simulink model "test_pi_flocking_gazebo"  (R2023b)
settings: Solver=FixedStepAuto  StartTime=0.0  StopTime=inf  RelTol=1e-3
values from neighbouring files (symbols this model uses):
  d_prime = 1    [main_flock3.m]    (also in main_flock4.m; params_flocking_ros.m)
  epsilon = 0.1    [main_flock3.m]    (also in main_flock4.m; params_flocking_ros.m)
  h = 0.2    [main_flock3.m]    (also in main_flock4.m; params_flocking_ros.m)
  R = 0.15    [main_flock3.m]    (also in main_flock4.m; params_flocking_ros.m)
  vxobs = 0    [main_flock3.m]    (also in main_flock4.m)
  vyobs = 0    [main_flock3.m]    (also in main_flock4.m)
  vzobs = 0    [main_flock3.m]    (also in main_flock4.m)
  xobs = 0.75    [main_flock3.m]    (also in main_flock4.m)
  yobs = -0.25    [main_flock3.m]    (also in main_flock4.m)
  zobs = 1.7    [main_flock3.m]    (also in main_flock4.m)
undefined symbols (not defined in the file or in its folder): angular, DiscIntNeverNeededParam, linear
libraries: ros2lib x14, simulink x4, robotcorelib x4
(part 1 of 2)
settings Model: Creator=johvany  LastModifiedBy=jonatan_alvarez
settings OptimizationCC: EnhancedBackFolding=on  PassReuseOutputArgsThreshold=0  ZeroExternalMemoryAtStartup=off  ZeroInternalMemoryAtStartup=off  MaxStackSize=64  OptimizeBlockOrder=speed  DifferentSizesBufferReuse=on  OptimizationCustomize=off
settings DebuggingCC: ParameterTunabilityLossMsg=error
settings HardwareCC: ProdBitPerLong=64  ProdHWDeviceType=Intel->x86-64 (Linux 64)  UseEmbeddedCoderFeatures=off
settings SFSimCC: MATLABDynamicMemAlloc=off
settings RTWCC: Description=Embedded Coder  SystemTargetFile=ert.tlc  HardwareBoard=Robot Operating System 2 (ROS 2)  TLCOptions="-aInlineSetEventsForThisBaseRateFcn=TLC_FALSE -aSuppressMultiTaskScheduler=TLC_FALSE  -aRateBasedStepFcn=0"  TemplateMakefile=ert_default_tmf  Toolchain=Colcon Tools  TargetLang=C++
settings CodeAppCC: ForceParamTrailComments=on  OperatorAnnotations=on
settings ERTTargetCC: ERTCustomFileBanners=off  CodeInterfacePackaging=C++ class  SupportContinuousTime=on  SupportNonInlinedSFcns=on  RemoveResetFunc=off  ModelStepFunctionPrototypeControlCompliant=off  RootIOFormat=Structure reference

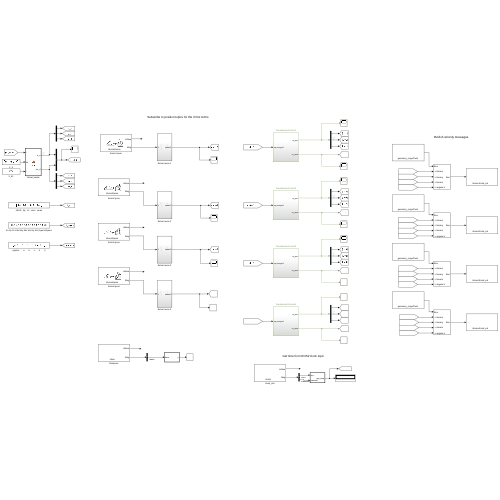
[thumbnail: Simulink's stored preview of the top-level diagram]
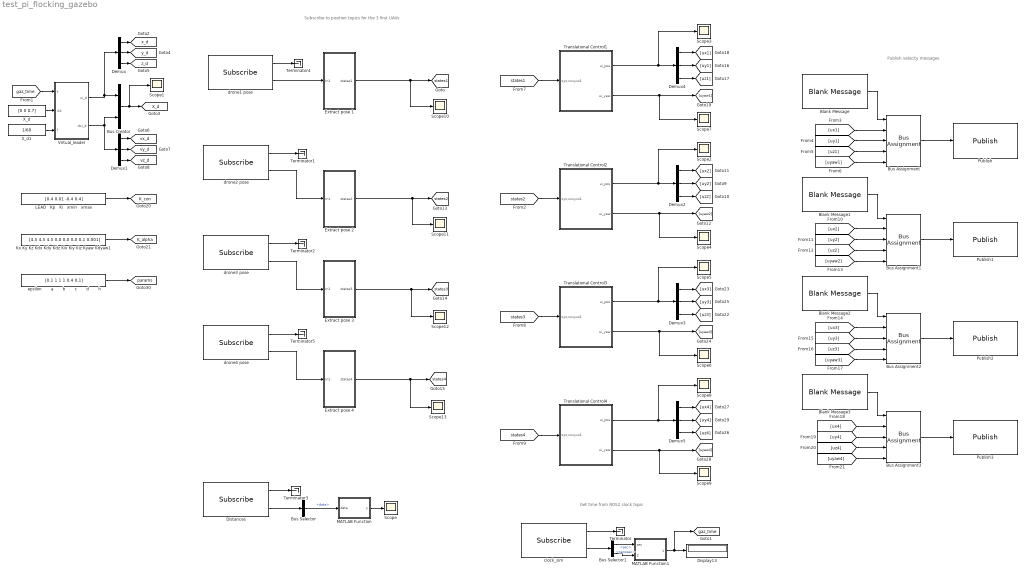
== system test_pi_flocking_gazebo ==
  note: Publish velocity messages
  note: Subscribe to position topics for the 3 first UAVs
  note: Get time from ROS2 clock topic
  Blank Message{,1..3} (4 alike) : ros2lib/Blank Message  messageClass=Message  entityType=geometry_msgs/Twist  messageType=geometry_msgs/Twist  SampleTime=inf
  Bus Assignment{,1..3} (4 alike) : BusAssignment  AssignedSignals=linear.x,linear.y,linear.z,angular.z
  Bus Creator : BusCreator  Inputs=2
  Bus Selector : BusSelector  OutputSignals=data
  Bus Selector1 : BusSelector  OutputSignals=clock.sec,clock.nanosec
  Demux{,1..5} (6 alike) : Demux  Outputs=3
  Display13 : Display
      settings: Decimation=4
  Distances : ros2lib/Subscribe  topicSource=Select from ROS network  topic=/dists  messageType=std_msgs/Float32MultiArray  sampleTime=-1  QOSHistory=Keep last  QOSDepth=1  QOSReliability=Reliable  QOSDurability=Volatile
  Extract pose 1 : Subsystem
  Extract pose 2 : Subsystem
  Extract pose 3 : Subsystem
  Extract pose 4 : Subsystem
  Kx Ky Kz Kdx Kdy Kdz Kix Kiy Kiz Kyaw Kdyaw1 : Constant  Value=[4.5 4.5 4.5 0.0 0.0 0.0 0.1 0.001]
  LEAD   Kp   Ki   xmin   xmax : Constant  Value=[0.4 0.01 -0.4 0.4]
  MATLAB Function : MATLAB Function  TreatAsAtomicUnit=on
  MATLAB Function1 : MATLAB Function  TreatAsAtomicUnit=on
  Publish : ros2lib/Publish  topicSource=Select from ROS network  topic=/drone1/cmd_vel  messageType=geometry_msgs/Twist  QOSHistory=Keep last  QOSDepth=1  QOSReliability=Reliable  QOSDurability=Volatile
  Publish1 : ros2lib/Publish  topicSource=Select from ROS network  topic=/drone2/cmd_vel  messageType=geometry_msgs/Twist  QOSHistory=Keep last  QOSDepth=1  QOSReliability=Reliable  QOSDurability=Volatile
  Publish2 : ros2lib/Publish  topicSource=Select from ROS network  topic=/drone3/cmd_vel  messageType=geometry_msgs/Twist  QOSHistory=Keep last  QOSDepth=1  QOSReliability=Reliable  QOSDurability=Volatile
  Publish3 : ros2lib/Publish  topicSource=Select from ROS network  topic=/drone4/cmd_vel  messageType=geometry_msgs/Twist  QOSHistory=Keep last  QOSDepth=1  QOSReliability=Reliable  QOSDurability=Volatile
  Scope{,1..13} (14 alike) : Scope
  Terminator{,1..5} (6 alike) : Terminator
  Translational Control1 : Subsystem
  Translational Control2 : Subsystem
  Translational Control3 : Subsystem
  Translational Control4 : Subsystem
  Virtual_leader : MATLAB Function  TreatAsAtomicUnit=on
  X_d : Constant  Value=[0 0 0.7]
  X_d1 : Constant  Value=1/60
  clock_sim : ros2lib/Subscribe  topicSource=Select from ROS network  topic=/clock  messageType=rosgraph_msgs/Clock  sampleTime=-1  QOSHistory=Keep last  QOSDepth=1  QOSReliability=Reliable  QOSDurability=Volatile
  drone1 pose : ros2lib/Subscribe  topicSource=Select from ROS network  topic=/drone1/pose  messageType=geometry_msgs/PoseStamped  sampleTime=-1  QOSHistory=Keep last  QOSDepth=1  QOSReliability=Reliable  QOSDurability=Volatile
  drone2 pose : ros2lib/Subscribe  topicSource=Select from ROS network  topic=/drone2/pose  messageType=geometry_msgs/PoseStamped  sampleTime=-1  QOSHistory=Keep last  QOSDepth=1  QOSReliability=Reliable  QOSDurability=Volatile
  drone3 pose : ros2lib/Subscribe  topicSource=Select from ROS network  topic=/drone3/pose  messageType=geometry_msgs/PoseStamped  sampleTime=-1  QOSHistory=Keep last  QOSDepth=1  QOSReliability=Reliable  QOSDurability=Volatile
  drone4 pose : ros2lib/Subscribe  topicSource=Select from ROS network  topic=/drone4/pose  messageType=geometry_msgs/PoseStamped  sampleTime=-1  QOSHistory=Keep last  QOSDepth=1  QOSReliability=Reliable  QOSDurability=Volatile
  epsilon       a       b       c       d       h : Constant  Value=[0.1 1 1 1 0.4 0.1]
  tag scope: K_alpha=global, K_con=global, X_d=global, gaz_time=global, params=global, states1=global, states2=global, states3=global, states4=global, vx_d=global, vy_d=global, vz_d=global, x_d=global, y_d=global, z_d=global
  wires:
  clock_sim/1 -> Terminator/1
  drone2 pose/2 -> Extract pose 2/1(In1)
  drone2 pose/1 -> Terminator1/1
  drone3 pose/2 -> Extract pose 3/1(In1)
  drone3 pose/1 -> Terminator2/1
  Blank Message/1 -> Bus Assignment/1
  Bus Assignment/1 -> Publish/1
  Blank Message1/1 -> Bus Assignment1/1
  Bus Assignment1/1 -> Publish1/1
  Blank Message2/1 -> Bus Assignment2/1
  Bus Assignment2/1 -> Publish2/1
  Blank Message3/1 -> Bus Assignment3/1
  Bus Assignment3/1 -> Publish3/1
  Distances/1 -> Terminator3/1
  Distances/2 -> Bus Selector/1
  Bus Selector/1 -> MATLAB Function/1(data)  "<data>"
  MATLAB Function/1(y) -> Scope/1
  clock_sim/2 -> Bus Selector1/1
  Bus Selector1/1 -> MATLAB Function1/1(sec)  "<sec>"
  Bus Selector1/2 -> MATLAB Function1/2(nanosec)  "<nanosec>"
  Demux1/1 -> [vx_d]
  Demux1/3 -> [vz_d]
  Demux/1 -> [x_d]
  Demux/2 -> [y_d]
  Virtual_leader/2(dxi_d) -> Bus Creator/2, Demux1/1
  Bus Creator/1 -> Scope1/1, [X_d]
  Demux1/2 -> [vy_d]
  [gaz_time] -> Virtual_leader/1(t)
  Demux/3 -> [z_d]
  Virtual_leader/1(xi_d) -> Bus Creator/1, Demux/1
  drone1 pose/1 -> Terminator4/1
  drone1 pose/2 -> Extract pose 1/1(In1)
  MATLAB Function1/1(gaz_time) -> [gaz_time], Display13/1
  Extract pose 1/1(states1) -> Scope10/1, [states1]
  [ux1] -> Bus Assignment/2
  [uy1] -> Bus Assignment/3
  [uz1] -> Bus Assignment/4
  [uyaw1] -> Bus Assignment/5
  X_d/1 -> Virtual_leader/2(Xd)
  Extract pose 2/1(states2) -> Scope11/1, [states2]
  Extract pose 3/1(states3) -> Scope12/1, [states3]
  drone4 pose/2 -> Extract pose 4/1(In1)
  drone4 pose/1 -> Terminator5/1
  Extract pose 4/1(states4) -> Scope13/1, [states4]
  [ux2] -> Bus Assignment1/2
  [uy2] -> Bus Assignment1/3
  [uz2] -> Bus Assignment1/4
  [uyaw2] -> Bus Assignment1/5
  [uy3] -> Bus Assignment2/3
  [uyaw3] -> Bus Assignment2/5
  [uz3] -> Bus Assignment2/4
  [ux3] -> Bus Assignment2/2
  [ux4] -> Bus Assignment3/2
  [uy4] -> Bus Assignment3/3
  [uz4] -> Bus Assignment3/4
  [uyaw4] -> Bus Assignment3/5
  Translational Control1/2(ui_yaw) -> [uyaw1], Scope7/1
  Demux4/2 -> [uy1]
  Demux4/3 -> [uz1]
  [states1] -> Translational Control1/1(xyz,vxvyvz1)
  Translational Control1/1(ui_pos) -> Scope3/1, Demux4/1
  Demux4/1 -> [ux1]
  LEAD   Kp   Ki   xmin   xmax/1 -> [K_con]
  Kx Ky Kz Kdx Kdy Kdz Kix Kiy Kiz Kyaw Kdyaw1/1 -> [K_alpha]
  Demux2/1 -> [ux2]
  Translational Control2/1(ui_pos) -> Demux2/1, Scope2/1
  [states2] -> Translational Control2/1(xyz,vxvyvz1)
  Demux2/3 -> [uz2]
  Demux2/2 -> [uy2]
  Translational Control2/2(ui_yaw) -> Scope4/1, [uyaw2]
  Translational Control3/2(ui_yaw) -> [uyaw3], Scope6/1
  Demux3/2 -> [uy3]
  Demux3/3 -> [uz3]
  [states3] -> Translational Control3/1(xyz,vxvyvz1)
  Translational Control3/1(ui_pos) -> Scope5/1, Demux3/1
  Demux3/1 -> [ux3]
  Demux5/1 -> [ux4]
  Translational Control4/1(ui_pos) -> Demux5/1, Scope8/1
  [states4] -> Translational Control4/1(xyz,vxvyvz1)
  Demux5/3 -> [uz4]
  Demux5/2 -> [uy4]
  Translational Control4/2(ui_yaw) -> Scope9/1, [uyaw4]
  epsilon       a       b       c       d       h/1 -> [params]
  X_d1/1 -> Virtual_leader/3(f)

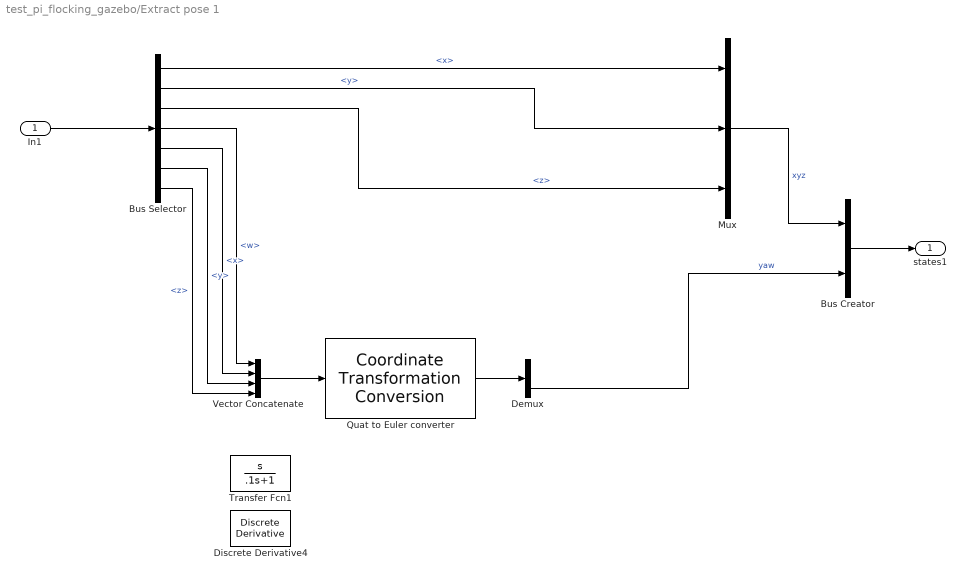
== system test_pi_flocking_gazebo/Extract pose 1 ==
  In1 : Inport
  Bus Creator : BusCreator  Inputs=2
  Bus Selector : BusSelector  OutputSignals=pose.position.x,pose.position.y,pose.position.z,pose.orientation.w,pose.orientation.x,pose.orientation.y,pose.orientation.z
  Demux : Demux  Outputs=3
  Discrete Derivative4 : simulink/Discrete/Discrete Derivative  gainval=1.0  ICPrevScaledInput=0.0  OutMin=[]  OutMax=[]  OutDataType=fixdt(1, 16)  OutScaling=2^-10  DoSatur=off
  Mux : Mux  Inputs=3
  Quat to Euler converter : robotcorelib/Coordinate Transformation Conversion  InputRepresentation=Quaternion  InputEulerSequence=ZYX  ShowTrVecInputPort=on  OutputRepresentation=Euler Angles  OutputEulerSequence=XYZ  ShowTrVecOutputPort=on  SimulateUsing=Interpreted execution
      settings: LibrarySourceBlock=roslib/Utilities/Coordinate Transformation Conversion
  Transfer Fcn1 : TransferFcn  Numerator=[1 0]  Denominator=[.1 1]
  Vector Concatenate : Concatenate  NumInputs=4
  states1 : Outport
  wires:
  Bus Selector/5 -> Vector Concatenate/2  "<x>"
  Quat to Euler converter/1 -> Demux/1
  Bus Selector/6 -> Vector Concatenate/3  "<y>"
  Bus Selector/1 -> Mux/1  "<x>"
  Bus Selector/7 -> Vector Concatenate/4  "<z>"
  Vector Concatenate/1 -> Quat to Euler converter/1
  In1/1 -> Bus Selector/1
  Bus Selector/4 -> Vector Concatenate/1  "<w>"
  Bus Selector/2 -> Mux/2  "<y>"
  Bus Selector/3 -> Mux/3  "<z>"
  Demux/3 -> Bus Creator/2  "yaw"
  Mux/1 -> Bus Creator/1  "xyz"
  Bus Creator/1 -> states1/1

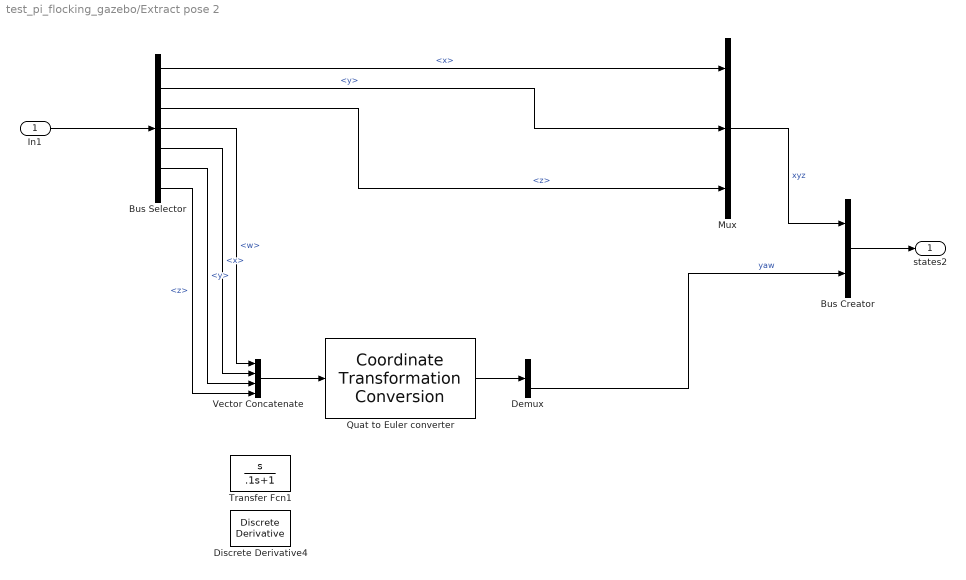
== system test_pi_flocking_gazebo/Extract pose 2 ==
  In1 : Inport
  Bus Creator : BusCreator  Inputs=2
  Bus Selector : BusSelector  OutputSignals=pose.position.x,pose.position.y,pose.position.z,pose.orientation.w,pose.orientation.x,pose.orientation.y,pose.orientation.z
  Demux : Demux  Outputs=3
  Discrete Derivative4 : simulink/Discrete/Discrete Derivative  gainval=1.0  ICPrevScaledInput=0.0  OutMin=[]  OutMax=[]  OutDataType=fixdt(1, 16)  OutScaling=2^-10  DoSatur=off
  Mux : Mux  Inputs=3
  Quat to Euler converter : robotcorelib/Coordinate Transformation Conversion  InputRepresentation=Quaternion  InputEulerSequence=ZYX  ShowTrVecInputPort=on  OutputRepresentation=Euler Angles  OutputEulerSequence=XYZ  ShowTrVecOutputPort=on  SimulateUsing=Interpreted execution
      settings: LibrarySourceBlock=roslib/Utilities/Coordinate Transformation Conversion
  Transfer Fcn1 : TransferFcn  Numerator=[1 0]  Denominator=[.1 1]
  Vector Concatenate : Concatenate  NumInputs=4
  states2 : Outport
  wires:
  Bus Creator/1 -> states2/1
  Mux/1 -> Bus Creator/1  "xyz"
  Demux/3 -> Bus Creator/2  "yaw"
  Bus Selector/3 -> Mux/3  "<z>"
  Bus Selector/2 -> Mux/2  "<y>"
  Bus Selector/4 -> Vector Concatenate/1  "<w>"
  In1/1 -> Bus Selector/1
  Vector Concatenate/1 -> Quat to Euler converter/1
  Bus Selector/7 -> Vector Concatenate/4  "<z>"
  Bus Selector/1 -> Mux/1  "<x>"
  Bus Selector/6 -> Vector Concatenate/3  "<y>"
  Quat to Euler converter/1 -> Demux/1
  Bus Selector/5 -> Vector Concatenate/2  "<x>"

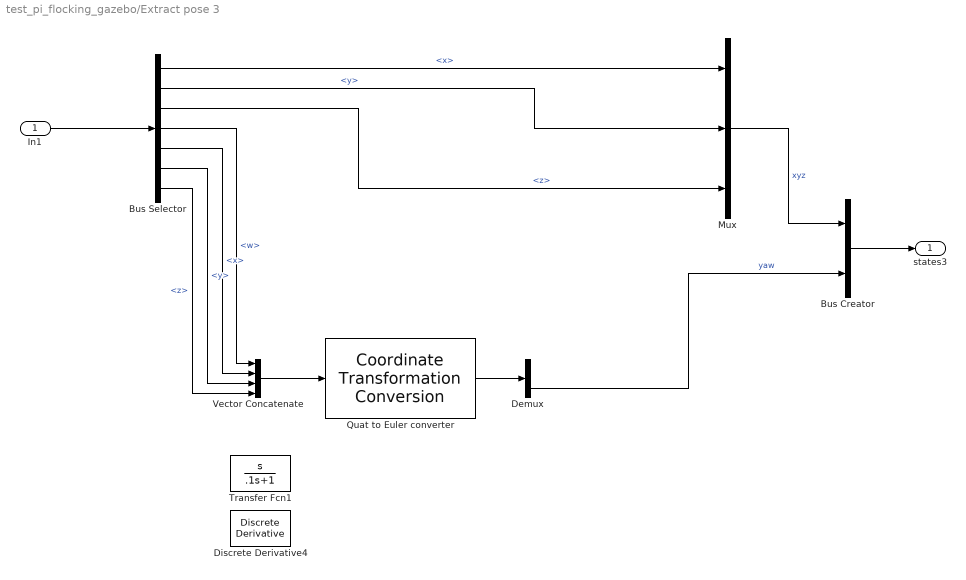
== system test_pi_flocking_gazebo/Extract pose 3 ==
  In1 : Inport
  Bus Creator : BusCreator  Inputs=2
  Bus Selector : BusSelector  OutputSignals=pose.position.x,pose.position.y,pose.position.z,pose.orientation.w,pose.orientation.x,pose.orientation.y,pose.orientation.z
  Demux : Demux  Outputs=3
  Discrete Derivative4 : simulink/Discrete/Discrete Derivative  gainval=1.0  ICPrevScaledInput=0.0  OutMin=[]  OutMax=[]  OutDataType=fixdt(1, 16)  OutScaling=2^-10  DoSatur=off
  Mux : Mux  Inputs=3
  Quat to Euler converter : robotcorelib/Coordinate Transformation Conversion  InputRepresentation=Quaternion  InputEulerSequence=ZYX  ShowTrVecInputPort=on  OutputRepresentation=Euler Angles  OutputEulerSequence=XYZ  ShowTrVecOutputPort=on  SimulateUsing=Interpreted execution
      settings: LibrarySourceBlock=roslib/Utilities/Coordinate Transformation Conversion
  Transfer Fcn1 : TransferFcn  Numerator=[1 0]  Denominator=[.1 1]
  Vector Concatenate : Concatenate  NumInputs=4
  states3 : Outport
  wires:
  Bus Selector/5 -> Vector Concatenate/2  "<x>"
  Quat to Euler converter/1 -> Demux/1
  Bus Selector/6 -> Vector Concatenate/3  "<y>"
  Bus Selector/1 -> Mux/1  "<x>"
  Bus Selector/7 -> Vector Concatenate/4  "<z>"
  Vector Concatenate/1 -> Quat to Euler converter/1
  In1/1 -> Bus Selector/1
  Bus Selector/4 -> Vector Concatenate/1  "<w>"
  Bus Selector/2 -> Mux/2  "<y>"
  Bus Selector/3 -> Mux/3  "<z>"
  Demux/3 -> Bus Creator/2  "yaw"
  Mux/1 -> Bus Creator/1  "xyz"
  Bus Creator/1 -> states3/1

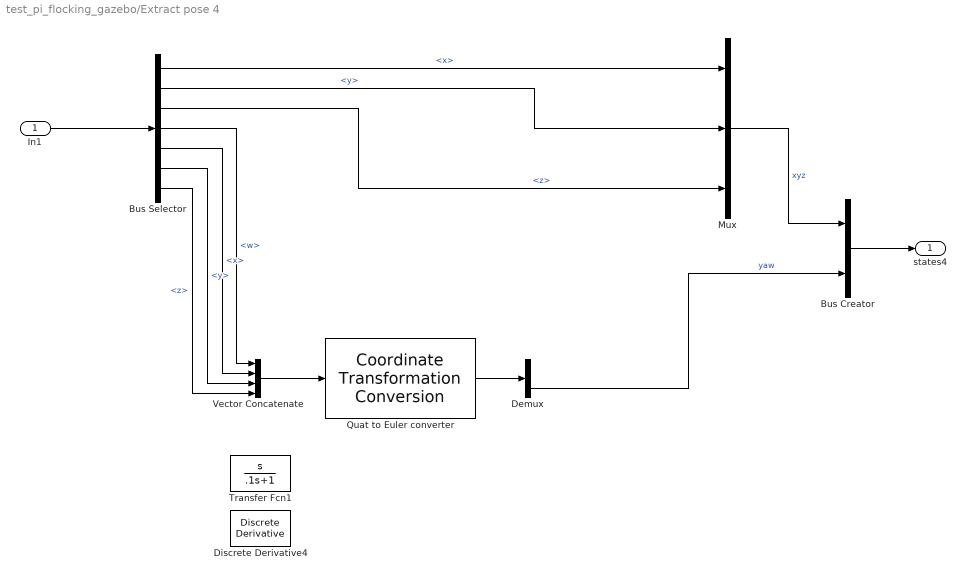
== system test_pi_flocking_gazebo/Extract pose 4 ==
  In1 : Inport
  Bus Creator : BusCreator  Inputs=2
  Bus Selector : BusSelector  OutputSignals=pose.position.x,pose.position.y,pose.position.z,pose.orientation.w,pose.orientation.x,pose.orientation.y,pose.orientation.z
  Demux : Demux  Outputs=3
  Discrete Derivative4 : simulink/Discrete/Discrete Derivative  gainval=1.0  ICPrevScaledInput=0.0  OutMin=[]  OutMax=[]  OutDataType=fixdt(1, 16)  OutScaling=2^-10  DoSatur=off
  Mux : Mux  Inputs=3
  Quat to Euler converter : robotcorelib/Coordinate Transformation Conversion  InputRepresentation=Quaternion  InputEulerSequence=ZYX  ShowTrVecInputPort=on  OutputRepresentation=Euler Angles  OutputEulerSequence=XYZ  ShowTrVecOutputPort=on  SimulateUsing=Interpreted execution
      settings: LibrarySourceBlock=roslib/Utilities/Coordinate Transformation Conversion
  Transfer Fcn1 : TransferFcn  Numerator=[1 0]  Denominator=[.1 1]
  Vector Concatenate : Concatenate  NumInputs=4
  states4 : Outport
  wires:
  Bus Creator/1 -> states4/1
  Mux/1 -> Bus Creator/1  "xyz"
  Demux/3 -> Bus Creator/2  "yaw"
  Bus Selector/3 -> Mux/3  "<z>"
  Bus Selector/2 -> Mux/2  "<y>"
  Bus Selector/4 -> Vector Concatenate/1  "<w>"
  In1/1 -> Bus Selector/1
  Vector Concatenate/1 -> Quat to Euler converter/1
  Bus Selector/7 -> Vector Concatenate/4  "<z>"
  Bus Selector/1 -> Mux/1  "<x>"
  Bus Selector/6 -> Vector Concatenate/3  "<y>"
  Quat to Euler converter/1 -> Demux/1
  Bus Selector/5 -> Vector Concatenate/2  "<x>"

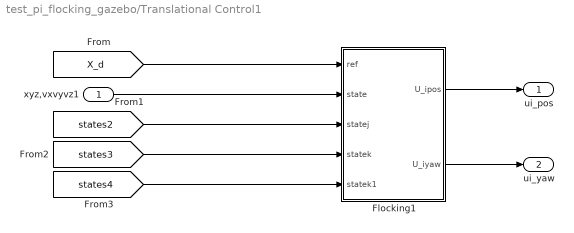
== system test_pi_flocking_gazebo/Translational Control1 ==
  xyz,vxvyvz1 : Inport
  Flocking1 : Subsystem
  ui_pos : Outport  VectorParamsAs1DForOutWhenUnconnected=off
  ui_yaw : Outport  Port=2  VectorParamsAs1DForOutWhenUnconnected=off
  wires:
  [X_d] -> Flocking1/1(ref)
  xyz,vxvyvz1/1 -> Flocking1/2(state)
  [states2] -> Flocking1/3(statej)
  [states3] -> Flocking1/4(statek)
  [states4] -> Flocking1/5(statek1)
  Flocking1/1(U_ipos) -> ui_pos/1
  Flocking1/2(U_iyaw) -> ui_yaw/1

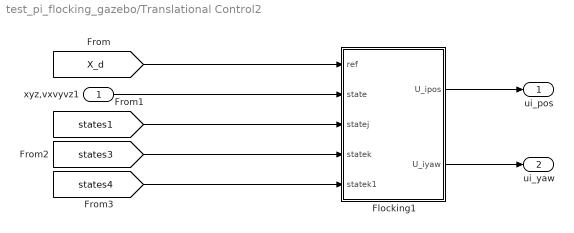
== system test_pi_flocking_gazebo/Translational Control2 ==
  xyz,vxvyvz1 : Inport
  Flocking1 : Subsystem
  ui_pos : Outport  VectorParamsAs1DForOutWhenUnconnected=off
  ui_yaw : Outport  Port=2  VectorParamsAs1DForOutWhenUnconnected=off
  wires:
  Flocking1/2(U_iyaw) -> ui_yaw/1
  Flocking1/1(U_ipos) -> ui_pos/1
  [states4] -> Flocking1/5(statek1)
  [states3] -> Flocking1/4(statek)
  [states1] -> Flocking1/3(statej)
  xyz,vxvyvz1/1 -> Flocking1/2(state)
  [X_d] -> Flocking1/1(ref)

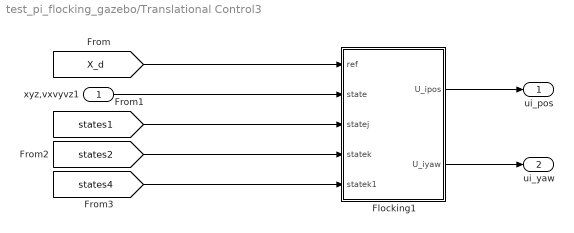
== system test_pi_flocking_gazebo/Translational Control3 ==
  xyz,vxvyvz1 : Inport
  Flocking1 : Subsystem
  ui_pos : Outport  VectorParamsAs1DForOutWhenUnconnected=off
  ui_yaw : Outport  Port=2  VectorParamsAs1DForOutWhenUnconnected=off
  wires:
  [X_d] -> Flocking1/1(ref)
  xyz,vxvyvz1/1 -> Flocking1/2(state)
  [states1] -> Flocking1/3(statej)
  [states2] -> Flocking1/4(statek)
  [states4] -> Flocking1/5(statek1)
  Flocking1/1(U_ipos) -> ui_pos/1
  Flocking1/2(U_iyaw) -> ui_yaw/1

== system test_pi_flocking_gazebo/Translational Control4 ==
  xyz,vxvyvz1 : Inport
  Flocking1 : Subsystem
  ui_pos : Outport  VectorParamsAs1DForOutWhenUnconnected=off
  ui_yaw : Outport  Port=2  VectorParamsAs1DForOutWhenUnconnected=off
  wires:
  Flocking1/2(U_iyaw) -> ui_yaw/1
  Flocking1/1(U_ipos) -> ui_pos/1
  [states3] -> Flocking1/5(statek1)
  [states2] -> Flocking1/4(statek)
  [states1] -> Flocking1/3(statej)
  xyz,vxvyvz1/1 -> Flocking1/2(state)
  [X_d] -> Flocking1/1(ref)

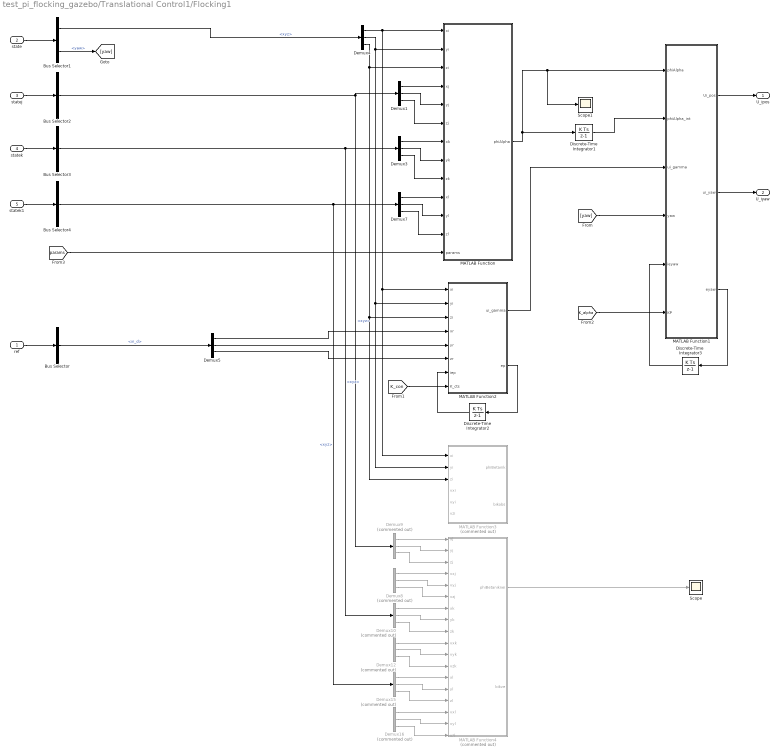
== system test_pi_flocking_gazebo/Translational Control1/Flocking1 ==
  ref : Inport
  state : Inport  Port=2
  statej : Inport  Port=3
  statek : Inport  Port=4
  statek1 : Inport  Port=5
  Bus Selector : BusSelector  OutputSignals=xi_d
  Bus Selector1 : BusSelector  OutputSignals=xyz,yaw
  Bus Selector2 : BusSelector  OutputSignals=xyz
  Bus Selector3 : BusSelector  OutputSignals=xyz
  Bus Selector4 : BusSelector  OutputSignals=xyz
  Demux{1,3..5,7} (5 alike) : Demux  Outputs=3
  Demux{8..10,12,15..16} (6 alike) : Demux  Commented=on  Outputs=3
  Discrete-Time Integrator1 : DiscreteIntegrator  SampleTime=-1  LimitOutput=on  UpperSaturationLimit=5  LowerSaturationLimit=-5  ICPrevOutput=DiscIntNeverNeededParam  ICPrevScaledInput=DiscIntNeverNeededParam
  Discrete-Time Integrator2 : DiscreteIntegrator  SampleTime=-1  LimitOutput=on  UpperSaturationLimit=2  LowerSaturationLimit=-2  ICPrevOutput=DiscIntNeverNeededParam  ICPrevScaledInput=DiscIntNeverNeededParam
  Discrete-Time Integrator3 : DiscreteIntegrator  SampleTime=-1  LimitOutput=on  UpperSaturationLimit=1  LowerSaturationLimit=-1  ICPrevOutput=DiscIntNeverNeededParam  ICPrevScaledInput=DiscIntNeverNeededParam
  MATLAB Function : MATLAB Function  TreatAsAtomicUnit=on
  MATLAB Function1 : MATLAB Function  TreatAsAtomicUnit=on
  MATLAB Function2 : MATLAB Function  TreatAsAtomicUnit=on
  MATLAB Function3 : MATLAB Function  Commented=on  TreatAsAtomicUnit=on
  MATLAB Function4 : MATLAB Function  Commented=on  TreatAsAtomicUnit=on
  Scope : Scope
  Scope1 : Scope
  U_ipos : Outport  VectorParamsAs1DForOutWhenUnconnected=off
  U_iyaw : Outport  Port=2  VectorParamsAs1DForOutWhenUnconnected=off
  wires:
  ref/1 -> Bus Selector/1
  state/1 -> Bus Selector1/1
  Bus Selector/1 -> Demux5/1  "<xi_d>"
  statej/1 -> Bus Selector2/1
  Bus Selector2/1 -> Demux1/1, Demux9/1  "<xyz>"
  Demux4/1 -> MATLAB Function/1(xi), MATLAB Function3/1(xi), MATLAB Function2/1(xi)
  Demux4/2 -> MATLAB Function/2(yi), MATLAB Function3/2(yi), MATLAB Function2/2(yi)
  Demux1/1 -> MATLAB Function/4(xj)
  Demux1/2 -> MATLAB Function/5(yj)
  Discrete-Time Integrator1/1 -> MATLAB Function1/2(phiAlpha_int)
  MATLAB Function2/1(ui_gamma) -> MATLAB Function1/3(ui_gamma)
  statek/1 -> Bus Selector3/1
  Demux3/1 -> MATLAB Function/7(xk)
  Demux3/2 -> MATLAB Function/8(yk)
  Bus Selector3/1 -> Demux10/1, Demux3/1  "<xyz>"
  Demux9/1 -> MATLAB Function4/1(xj)
  Demux9/2 -> MATLAB Function4/2(yj)
  Demux10/1 -> MATLAB Function4/7(xk)
  Demux10/2 -> MATLAB Function4/8(yk)
  MATLAB Function/1(phiAlpha) -> Scope1/1, MATLAB Function1/1(phiAlpha), Discrete-Time Integrator1/1
  Demux5/1 -> MATLAB Function2/4(xr)
  Demux5/2 -> MATLAB Function2/5(yr)
  Demux4/3 -> MATLAB Function/3(zi), MATLAB Function3/3(zi), MATLAB Function2/3(zi)
  Demux3/3 -> MATLAB Function/9(zk)
  Demux5/3 -> MATLAB Function2/6(zr)
  MATLAB Function1/1(Ui_pos) -> U_ipos/1
  Demux1/3 -> MATLAB Function/6(zj)
  Demux9/3 -> MATLAB Function4/3(zj)
  Demux10/3 -> MATLAB Function4/9(zk)
  MATLAB Function4/1(phiBetaniknei) -> Scope/1
  Demux8/1 -> MATLAB Function4/4(vxj)
  Demux8/2 -> MATLAB Function4/5(vyj)
  Demux8/3 -> MATLAB Function4/6(vzj)
  Demux12/1 -> MATLAB Function4/10(vxk)
  Demux12/2 -> MATLAB Function4/11(vyk)
  Demux12/3 -> MATLAB Function4/12(vzk)
  statek1/1 -> Bus Selector4/1
  Demux7/1 -> MATLAB Function/10(xl)
  Demux7/2 -> MATLAB Function/11(yl)
  Demux7/3 -> MATLAB Function/12(zl)
  Bus Selector4/1 -> Demux15/1, Demux7/1  "<xyz>"
  Demux15/1 -> MATLAB Function4/13(xl)
  Demux15/2 -> MATLAB Function4/14(yl)
  Demux15/3 -> MATLAB Function4/15(zl)
  Demux16/1 -> MATLAB Function4/16(vxl)
  Demux16/2 -> MATLAB Function4/17(vyl)
  Demux16/3 -> MATLAB Function4/18(vzl)
  Bus Selector1/1 -> Demux4/1  "<xyz>"
  Bus Selector1/2 -> [yaw]  "<yaw>"
  [yaw] -> MATLAB Function1/4(yaw)
  MATLAB Function1/2(ui_yaw) -> U_iyaw/1
  MATLAB Function2/2(ep) -> Discrete-Time Integrator2/1
  Discrete-Time Integrator2/1 -> MATLAB Function2/7(iep)
  [K_con] -> MATLAB Function2/8(K_cts)
  MATLAB Function1/3(eyaw) -> Discrete-Time Integrator3/1
  Discrete-Time Integrator3/1 -> MATLAB Function1/5(ieyaw)
  [K_alpha] -> MATLAB Function1/6(KP)
  [params] -> MATLAB Function/13(params)

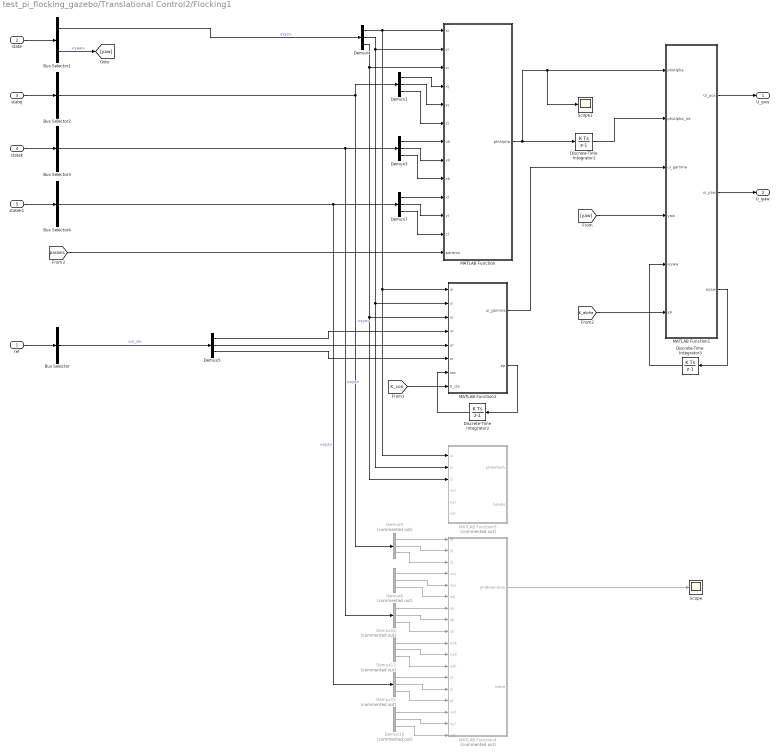
== system test_pi_flocking_gazebo/Translational Control2/Flocking1 ==
  ref : Inport
  state : Inport  Port=2
  statej : Inport  Port=3
  statek : Inport  Port=4
  statek1 : Inport  Port=5
  Bus Selector : BusSelector  OutputSignals=xi_d
  Bus Selector1 : BusSelector  OutputSignals=xyz,yaw
  Bus Selector2 : BusSelector  OutputSignals=xyz
  Bus Selector3 : BusSelector  OutputSignals=xyz
  Bus Selector4 : BusSelector  OutputSignals=xyz
  Demux{1,3..5,7} (5 alike) : Demux  Outputs=3
  Demux{8..10,12,15..16} (6 alike) : Demux  Commented=on  Outputs=3
  Discrete-Time Integrator1 : DiscreteIntegrator  SampleTime=-1  LimitOutput=on  UpperSaturationLimit=5  LowerSaturationLimit=-5  ICPrevOutput=DiscIntNeverNeededParam  ICPrevScaledInput=DiscIntNeverNeededParam
  Discrete-Time Integrator2 : DiscreteIntegrator  SampleTime=-1  LimitOutput=on  UpperSaturationLimit=2  LowerSaturationLimit=-2  ICPrevOutput=DiscIntNeverNeededParam  ICPrevScaledInput=DiscIntNeverNeededParam
  Discrete-Time Integrator3 : DiscreteIntegrator  SampleTime=-1  LimitOutput=on  UpperSaturationLimit=1  LowerSaturationLimit=-1  ICPrevOutput=DiscIntNeverNeededParam  ICPrevScaledInput=DiscIntNeverNeededParam
  MATLAB Function : MATLAB Function  TreatAsAtomicUnit=on
  MATLAB Function1 : MATLAB Function  TreatAsAtomicUnit=on
  MATLAB Function2 : MATLAB Function  TreatAsAtomicUnit=on
  MATLAB Function3 : MATLAB Function  Commented=on  TreatAsAtomicUnit=on
  MATLAB Function4 : MATLAB Function  Commented=on  TreatAsAtomicUnit=on
  Scope : Scope
  Scope1 : Scope
  U_ipos : Outport  VectorParamsAs1DForOutWhenUnconnected=off
  U_iyaw : Outport  Port=2  VectorParamsAs1DForOutWhenUnconnected=off
  wires:
  [K_alpha] -> MATLAB Function1/6(KP)
  Discrete-Time Integrator3/1 -> MATLAB Function1/5(ieyaw)
  MATLAB Function1/3(eyaw) -> Discrete-Time Integrator3/1
  [K_con] -> MATLAB Function2/8(K_cts)
  Discrete-Time Integrator2/1 -> MATLAB Function2/7(iep)
  MATLAB Function2/2(ep) -> Discrete-Time Integrator2/1
  MATLAB Function1/2(ui_yaw) -> U_iyaw/1
  [yaw] -> MATLAB Function1/4(yaw)
  Bus Selector1/2 -> [yaw]  "<yaw>"
  Bus Selector1/1 -> Demux4/1  "<xyz>"
  Demux16/3 -> MATLAB Function4/18(vzl)
  Demux16/2 -> MATLAB Function4/17(vyl)
  Demux16/1 -> MATLAB Function4/16(vxl)
  Demux15/3 -> MATLAB Function4/15(zl)
  Demux15/2 -> MATLAB Function4/14(yl)
  Demux15/1 -> MATLAB Function4/13(xl)
  Bus Selector4/1 -> Demux7/1, Demux15/1  "<xyz>"
  Demux7/3 -> MATLAB Function/12(zl)
  Demux7/2 -> MATLAB Function/11(yl)
  Demux7/1 -> MATLAB Function/10(xl)
  statek1/1 -> Bus Selector4/1
  Demux12/3 -> MATLAB Function4/12(vzk)
  Demux12/2 -> MATLAB Function4/11(vyk)
  Demux12/1 -> MATLAB Function4/10(vxk)
  Demux8/3 -> MATLAB Function4/6(vzj)
  Demux8/2 -> MATLAB Function4/5(vyj)
  Demux8/1 -> MATLAB Function4/4(vxj)
  MATLAB Function4/1(phiBetaniknei) -> Scope/1
  Demux10/3 -> MATLAB Function4/9(zk)
  Demux9/3 -> MATLAB Function4/3(zj)
  Demux1/3 -> MATLAB Function/6(zj)
  MATLAB Function1/1(Ui_pos) -> U_ipos/1
  Demux5/3 -> MATLAB Function2/6(zr)
  Demux3/3 -> MATLAB Function/9(zk)
  Demux4/3 -> MATLAB Function/3(zi), MATLAB Function2/3(zi), MATLAB Function3/3(zi)
  Demux5/2 -> MATLAB Function2/5(yr)
  Demux5/1 -> MATLAB Function2/4(xr)
  MATLAB Function/1(phiAlpha) -> MATLAB Function1/1(phiAlpha), Scope1/1, Discrete-Time Integrator1/1
  Demux10/2 -> MATLAB Function4/8(yk)
  Demux10/1 -> MATLAB Function4/7(xk)
  Demux9/2 -> MATLAB Function4/2(yj)
  Demux9/1 -> MATLAB Function4/1(xj)
  Bus Selector3/1 -> Demux3/1, Demux10/1  "<xyz>"
  Demux3/2 -> MATLAB Function/8(yk)
  Demux3/1 -> MATLAB Function/7(xk)
  statek/1 -> Bus Selector3/1
  MATLAB Function2/1(ui_gamma) -> MATLAB Function1/3(ui_gamma)
  Discrete-Time Integrator1/1 -> MATLAB Function1/2(phiAlpha_int)
  Demux1/2 -> MATLAB Function/5(yj)
  Demux1/1 -> MATLAB Function/4(xj)
  Demux4/2 -> MATLAB Function/2(yi), MATLAB Function2/2(yi), MATLAB Function3/2(yi)
  Demux4/1 -> MATLAB Function/1(xi), MATLAB Function2/1(xi), MATLAB Function3/1(xi)
  Bus Selector2/1 -> Demux9/1, Demux1/1  "<xyz>"
  statej/1 -> Bus Selector2/1
  Bus Selector/1 -> Demux5/1  "<xi_d>"
  state/1 -> Bus Selector1/1
  ref/1 -> Bus Selector/1
  [params] -> MATLAB Function/13(params)

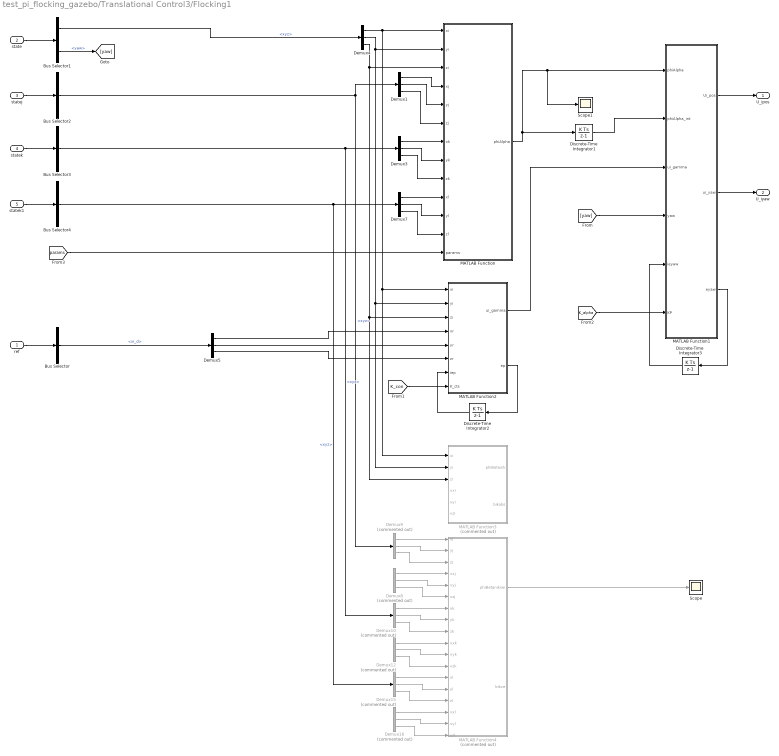
== system test_pi_flocking_gazebo/Translational Control3/Flocking1 ==
  ref : Inport
  state : Inport  Port=2
  statej : Inport  Port=3
  statek : Inport  Port=4
  statek1 : Inport  Port=5
  Bus Selector : BusSelector  OutputSignals=xi_d
  Bus Selector1 : BusSelector  OutputSignals=xyz,yaw
  Bus Selector2 : BusSelector  OutputSignals=xyz
  Bus Selector3 : BusSelector  OutputSignals=xyz
  Bus Selector4 : BusSelector  OutputSignals=xyz
  Demux{1,3..5,7} (5 alike) : Demux  Outputs=3
  Demux{8..10,12,15..16} (6 alike) : Demux  Commented=on  Outputs=3
  Discrete-Time Integrator1 : DiscreteIntegrator  SampleTime=-1  LimitOutput=on  UpperSaturationLimit=5  LowerSaturationLimit=-5  ICPrevOutput=DiscIntNeverNeededParam  ICPrevScaledInput=DiscIntNeverNeededParam
  Discrete-Time Integrator2 : DiscreteIntegrator  SampleTime=-1  LimitOutput=on  UpperSaturationLimit=2  LowerSaturationLimit=-2  ICPrevOutput=DiscIntNeverNeededParam  ICPrevScaledInput=DiscIntNeverNeededParam
  Discrete-Time Integrator3 : DiscreteIntegrator  SampleTime=-1  LimitOutput=on  UpperSaturationLimit=1  LowerSaturationLimit=-1  ICPrevOutput=DiscIntNeverNeededParam  ICPrevScaledInput=DiscIntNeverNeededParam
  MATLAB Function : MATLAB Function  TreatAsAtomicUnit=on
  MATLAB Function1 : MATLAB Function  TreatAsAtomicUnit=on
  MATLAB Function2 : MATLAB Function  TreatAsAtomicUnit=on
  MATLAB Function3 : MATLAB Function  Commented=on  TreatAsAtomicUnit=on
  MATLAB Function4 : MATLAB Function  Commented=on  TreatAsAtomicUnit=on
  Scope : Scope
  Scope1 : Scope
  U_ipos : Outport  VectorParamsAs1DForOutWhenUnconnected=off
  U_iyaw : Outport  Port=2  VectorParamsAs1DForOutWhenUnconnected=off
  wires:
  ref/1 -> Bus Selector/1
  state/1 -> Bus Selector1/1
  Bus Selector/1 -> Demux5/1  "<xi_d>"
  statej/1 -> Bus Selector2/1
  Bus Selector2/1 -> Demux1/1, Demux9/1  "<xyz>"
  Demux4/1 -> MATLAB Function/1(xi), MATLAB Function2/1(xi), MATLAB Function3/1(xi)
  Demux4/2 -> MATLAB Function/2(yi), MATLAB Function2/2(yi), MATLAB Function3/2(yi)
  Demux1/1 -> MATLAB Function/4(xj)
  Demux1/2 -> MATLAB Function/5(yj)
  Discrete-Time Integrator1/1 -> MATLAB Function1/2(phiAlpha_int)
  MATLAB Function2/1(ui_gamma) -> MATLAB Function1/3(ui_gamma)
  statek/1 -> Bus Selector3/1
  Demux3/1 -> MATLAB Function/7(xk)
  Demux3/2 -> MATLAB Function/8(yk)
  Bus Selector3/1 -> Demux10/1, Demux3/1  "<xyz>"
  Demux9/1 -> MATLAB Function4/1(xj)
  Demux9/2 -> MATLAB Function4/2(yj)
  Demux10/1 -> MATLAB Function4/7(xk)
  Demux10/2 -> MATLAB Function4/8(yk)
  MATLAB Function/1(phiAlpha) -> Scope1/1, MATLAB Function1/1(phiAlpha), Discrete-Time Integrator1/1
  Demux5/1 -> MATLAB Function2/4(xr)
  Demux5/2 -> MATLAB Function2/5(yr)
  Demux4/3 -> MATLAB Function/3(zi), MATLAB Function2/3(zi), MATLAB Function3/3(zi)
  Demux3/3 -> MATLAB Function/9(zk)
  Demux5/3 -> MATLAB Function2/6(zr)
  MATLAB Function1/1(Ui_pos) -> U_ipos/1
  Demux1/3 -> MATLAB Function/6(zj)
  Demux9/3 -> MATLAB Function4/3(zj)
  Demux10/3 -> MATLAB Function4/9(zk)
  MATLAB Function4/1(phiBetaniknei) -> Scope/1
  Demux8/1 -> MATLAB Function4/4(vxj)
  Demux8/2 -> MATLAB Function4/5(vyj)
  Demux8/3 -> MATLAB Function4/6(vzj)
  Demux12/1 -> MATLAB Function4/10(vxk)
  Demux12/2 -> MATLAB Function4/11(vyk)
  Demux12/3 -> MATLAB Function4/12(vzk)
  statek1/1 -> Bus Selector4/1
  Demux7/1 -> MATLAB Function/10(xl)
  Demux7/2 -> MATLAB Function/11(yl)
  Demux7/3 -> MATLAB Function/12(zl)
  Bus Selector4/1 -> Demux15/1, Demux7/1  "<xyz>"
  Demux15/1 -> MATLAB Function4/13(xl)
  Demux15/2 -> MATLAB Function4/14(yl)
  Demux15/3 -> MATLAB Function4/15(zl)
  Demux16/1 -> MATLAB Function4/16(vxl)
  Demux16/2 -> MATLAB Function4/17(vyl)
  Demux16/3 -> MATLAB Function4/18(vzl)
  Bus Selector1/1 -> Demux4/1  "<xyz>"
  Bus Selector1/2 -> [yaw]  "<yaw>"
  [yaw] -> MATLAB Function1/4(yaw)
  MATLAB Function1/2(ui_yaw) -> U_iyaw/1
  MATLAB Function2/2(ep) -> Discrete-Time Integrator2/1
  Discrete-Time Integrator2/1 -> MATLAB Function2/7(iep)
  [K_con] -> MATLAB Function2/8(K_cts)
  MATLAB Function1/3(eyaw) -> Discrete-Time Integrator3/1
  Discrete-Time Integrator3/1 -> MATLAB Function1/5(ieyaw)
  [K_alpha] -> MATLAB Function1/6(KP)
  [params] -> MATLAB Function/13(params)

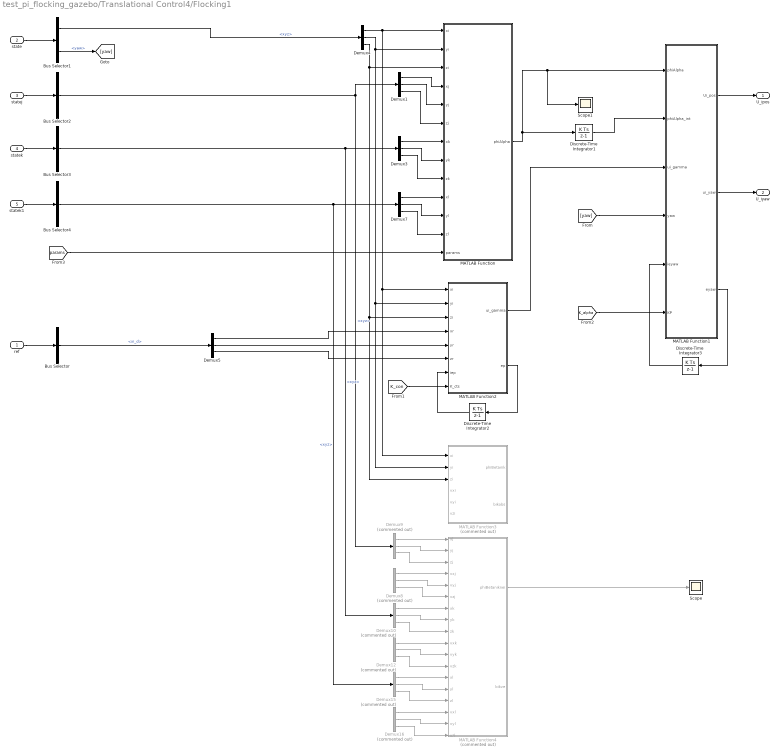
== system test_pi_flocking_gazebo/Translational Control4/Flocking1 ==
  ref : Inport
  state : Inport  Port=2
  statej : Inport  Port=3
  statek : Inport  Port=4
  statek1 : Inport  Port=5
  Bus Selector : BusSelector  OutputSignals=xi_d
  Bus Selector1 : BusSelector  OutputSignals=xyz,yaw
  Bus Selector2 : BusSelector  OutputSignals=xyz
  Bus Selector3 : BusSelector  OutputSignals=xyz
  Bus Selector4 : BusSelector  OutputSignals=xyz
  Demux{1,3..5,7} (5 alike) : Demux  Outputs=3
  Demux{8..10,12,15..16} (6 alike) : Demux  Commented=on  Outputs=3
  Discrete-Time Integrator1 : DiscreteIntegrator  SampleTime=-1  LimitOutput=on  UpperSaturationLimit=5  LowerSaturationLimit=-5  ICPrevOutput=DiscIntNeverNeededParam  ICPrevScaledInput=DiscIntNeverNeededParam
  Discrete-Time Integrator2 : DiscreteIntegrator  SampleTime=-1  LimitOutput=on  UpperSaturationLimit=2  LowerSaturationLimit=-2  ICPrevOutput=DiscIntNeverNeededParam  ICPrevScaledInput=DiscIntNeverNeededParam
  Discrete-Time Integrator3 : DiscreteIntegrator  SampleTime=-1  LimitOutput=on  UpperSaturationLimit=1  LowerSaturationLimit=-1  ICPrevOutput=DiscIntNeverNeededParam  ICPrevScaledInput=DiscIntNeverNeededParam
  MATLAB Function : MATLAB Function  TreatAsAtomicUnit=on
  MATLAB Function1 : MATLAB Function  TreatAsAtomicUnit=on
  MATLAB Function2 : MATLAB Function  TreatAsAtomicUnit=on
  MATLAB Function3 : MATLAB Function  Commented=on  TreatAsAtomicUnit=on
  MATLAB Function4 : MATLAB Function  Commented=on  TreatAsAtomicUnit=on
  Scope : Scope
  Scope1 : Scope
  U_ipos : Outport  VectorParamsAs1DForOutWhenUnconnected=off
  U_iyaw : Outport  Port=2  VectorParamsAs1DForOutWhenUnconnected=off
  wires:
  [K_alpha] -> MATLAB Function1/6(KP)
  Discrete-Time Integrator3/1 -> MATLAB Function1/5(ieyaw)
  MATLAB Function1/3(eyaw) -> Discrete-Time Integrator3/1
  [K_con] -> MATLAB Function2/8(K_cts)
  Discrete-Time Integrator2/1 -> MATLAB Function2/7(iep)
  MATLAB Function2/2(ep) -> Discrete-Time Integrator2/1
  MATLAB Function1/2(ui_yaw) -> U_iyaw/1
  [yaw] -> MATLAB Function1/4(yaw)
  Bus Selector1/2 -> [yaw]  "<yaw>"
  Bus Selector1/1 -> Demux4/1  "<xyz>"
  Demux16/3 -> MATLAB Function4/18(vzl)
  Demux16/2 -> MATLAB Function4/17(vyl)
  Demux16/1 -> MATLAB Function4/16(vxl)
  Demux15/3 -> MATLAB Function4/15(zl)
  Demux15/2 -> MATLAB Function4/14(yl)
  Demux15/1 -> MATLAB Function4/13(xl)
  Bus Selector4/1 -> Demux7/1, Demux15/1  "<xyz>"
  Demux7/3 -> MATLAB Function/12(zl)
  Demux7/2 -> MATLAB Function/11(yl)
  Demux7/1 -> MATLAB Function/10(xl)
  statek1/1 -> Bus Selector4/1
  Demux12/3 -> MATLAB Function4/12(vzk)
  Demux12/2 -> MATLAB Function4/11(vyk)
  Demux12/1 -> MATLAB Function4/10(vxk)
  Demux8/3 -> MATLAB Function4/6(vzj)
  Demux8/2 -> MATLAB Function4/5(vyj)
  Demux8/1 -> MATLAB Function4/4(vxj)
  MATLAB Function4/1(phiBetaniknei) -> Scope/1
  Demux10/3 -> MATLAB Function4/9(zk)
  Demux9/3 -> MATLAB Function4/3(zj)
  Demux1/3 -> MATLAB Function/6(zj)
  MATLAB Function1/1(Ui_pos) -> U_ipos/1
  Demux5/3 -> MATLAB Function2/6(zr)
  Demux3/3 -> MATLAB Function/9(zk)
  Demux4/3 -> MATLAB Function/3(zi), MATLAB Function2/3(zi), MATLAB Function3/3(zi)
  Demux5/2 -> MATLAB Function2/5(yr)
  Demux5/1 -> MATLAB Function2/4(xr)
  MATLAB Function/1(phiAlpha) -> Discrete-Time Integrator1/1, MATLAB Function1/1(phiAlpha), Scope1/1
  Demux10/2 -> MATLAB Function4/8(yk)
  Demux10/1 -> MATLAB Function4/7(xk)
  Demux9/2 -> MATLAB Function4/2(yj)
  Demux9/1 -> MATLAB Function4/1(xj)
  Bus Selector3/1 -> Demux3/1, Demux10/1  "<xyz>"
  Demux3/2 -> MATLAB Function/8(yk)
  Demux3/1 -> MATLAB Function/7(xk)
  statek/1 -> Bus Selector3/1
  MATLAB Function2/1(ui_gamma) -> MATLAB Function1/3(ui_gamma)
  Discrete-Time Integrator1/1 -> MATLAB Function1/2(phiAlpha_int)
  Demux1/2 -> MATLAB Function/5(yj)
  Demux1/1 -> MATLAB Function/4(xj)
  Demux4/2 -> MATLAB Function/2(yi), MATLAB Function2/2(yi), MATLAB Function3/2(yi)
  Demux4/1 -> MATLAB Function/1(xi), MATLAB Function2/1(xi), MATLAB Function3/1(xi)
  Bus Selector2/1 -> Demux9/1, Demux1/1  "<xyz>"
  statej/1 -> Bus Selector2/1
  Bus Selector/1 -> Demux5/1  "<xi_d>"
  state/1 -> Bus Selector1/1
  ref/1 -> Bus Selector/1
  [params] -> MATLAB Function/13(params)

== matlab function test_pi_flocking_gazebo/MATLAB Function ==
  data: data input; y output
function y = fcn(data)

DATA = data(1:20);
d1 = DATA(1);
d2 = DATA(2);
d3 = DATA(3);
y = [d1;d2;d3];

== matlab function test_pi_flocking_gazebo/Virtual_leader ==
  data: t input; xi_d output; dxi_d output; Xd input; f input
function [xi_d, dxi_d]  = fcn(t, Xd, f)
%#codegen



%f=1/60;    %freq in Hz
radius=1;   %radius in meters
f2 = 1/35;
radius2 = 1;
sel=2;      %inputs or parameters dont work! only local vars ...

if sel == 1
    if t < 90
       xd     =  0;
       xdotd  =  0;
           
       yd     = 0;
       ydotd  = 0;
           
       zd     = 0.7;  
       zdotd  = 0; 
           
       xi_d =[xd; yd; zd];
       dxi_d=[xdotd; ydotd; zdotd]; 
       
    elseif t < 120
        xd     =  0.4;
        xdotd  =  0;
            
        yd     = -0.4;
        ydotd  = 0;
            
        zd     = 0.7;  
        zdotd  = 0; 
            
        xi_d =[xd; yd; zd];
        dxi_d=[xdotd; ydotd; zdotd]; 
        
    else
       xd     = radius*sin(2*pi*f*t);
       xdotd  = radius*2*pi*f*cos(2*pi*f*t);
            
       yd     = radius*cos(2*pi*f*t);
       ydotd  = -radius*2*pi*f*sin(2*pi*f*t);
            
       zd     = 0.7;  %radius*cos(2*pi*f*t) + 5;
       zdotd  = 0;  %-radius*2*pi*f*sin(2*pi*f*t);
           
       xi_d =[xd; yd; zd];
       dxi_d=[xdotd; ydotd; zdotd];
       
    end
end

 if(sel==2)
     xd     =  Xd(1);
     xdotd  =  0;
          
     yd     = Xd(2);
     ydotd  = 0;
          
     zd     = Xd(3);  
     zdotd  = 0; 
          
     xi_d =[xd; yd; zd];
     dxi_d=[xdotd; ydotd; zdotd]; 
     
 end

== matlab function test_pi_flocking_gazebo/Translational Control2/Flocking1/MATLAB Function ==
  data: xi input; yi input; zi input; phiAlpha output; xj input; yj input; zj input; xk input; yk input; zk input; xl input; yl input; zl input; params input

function phiAlpha  = phiAlphaFcn(xi, yi, zi, xj, yj, zj, xk, yk, zk, xl, yl, zl, params)
    
    % Flocking parameters
    epsilon = params(1); a = params(2); b = params(3); c = params(4); d = params(5); h = params(6);

    e = abs(a - b) / sqrt(4*a*b) ;

    cAlpha = sigmaNormFun(c, epsilon) ;
    dAlpha = sigmaNormFun(d, epsilon) ;

    %%
    Pi = [xi;yi;zi] ;
    Pj = [xj;yj;zj] ;
    Pk = [xk;yk;zk] ;
    Pl = [xl;yl;zl] ;

    %%
    sigmaNormj = sigmaNormFun(Pj - Pi, epsilon) ;
    nij = gradSigmaFun(Pj - Pi, epsilon) ;
    
    sigmaNormk = sigmaNormFun(Pk - Pi, epsilon) ;
    nik = gradSigmaFun(Pk - Pi, epsilon) ;

    sigmaNorml = sigmaNormFun(Pl - Pi, epsilon) ;
    nil = gradSigmaFun(Pl - Pi, epsilon) ;

    %%
    sigma1j = sigma1Fun(sigmaNormj - dAlpha + e) ;
    sigma1k = sigma1Fun(sigmaNormk - dAlpha + e) ;
    sigma1l = sigma1Fun(sigmaNorml - dAlpha + e) ;
            
    %% Position
    phiAlphaj = 0.5 * bumpFcn(sigmaNormj/cAlpha,h) * ((a+b)*sigma1j + (a-b)) ;
    phiAlphanij = phiAlphaj.* nij ;
    
    phiAlphak = 0.5 * bumpFcn(sigmaNormk/cAlpha,h) * ((a+b)*sigma1k + (a-b)) ;
    phiAlphanik = phiAlphak.* nik ;

    phiAlphal = 0.5 * bumpFcn(sigmaNorml/cAlpha,h) * ((a+b)*sigma1l + (a-b)) ;
    phiAlphanil = phiAlphal.* nil ;

    phiAlpha = phiAlphanij + phiAlphanik + phiAlphanil;

    
end

== matlab function test_pi_flocking_gazebo/Translational Control2/Flocking1/MATLAB Function1 ==
  data: phiAlpha input; phiAlpha_int input; ui_gamma input; yaw input; ieyaw input; Ui_pos output size=3; ui_yaw output; KP input; eyaw output

function [Ui_pos, ui_yaw, eyaw]  = ctrlLaw(phiAlpha, phiAlpha_int, ui_gamma, yaw, ieyaw, KP)  %, phiBetak, bikobs, phiBetanei, bikve
    
    % Control gains and parameters
    Kx = KP(1); Ky = KP(2); Kz = KP(3);
    Kix = KP(4); Kiy = KP(5); Kiz = KP(6);
    Kyaw = KP(8); Kiyaw = KP(7);
    
    hx_dot = Kx * phiAlpha(1,1) + Kix * phiAlpha_int(1,1) + ui_gamma(1,1);  %+ cBetax * (phiBetak(1,1) + phiBetanei(1,1)) + cdBetax * (bikobs(1,1) + bikve(1,1));
    hy_dot = Ky * phiAlpha(2,1) + Kiy * phiAlpha_int(2,1) + ui_gamma(2,1);  %+ cBetay * (phiBetak(2,1) + phiBetanei(2,1)) + cdBetay * (bikobs(2,1) + bikve(2,1));
    hz_dot = Kz * phiAlpha(3,1) + Kiz * phiAlpha_int(3,1) + ui_gamma(3,1);  %+ cBetaz * (phiBetak(3,1) + phiBetanei(3,1)) + cdBetaz * (bikobs(3,1) + bikve(3,1));
    

    eyaw = 0 - yaw;
    

    Ui_pos = [hx_dot; hy_dot; hz_dot] ;
    ui_yaw = Kyaw*eyaw + Kiyaw*ieyaw;

end

== matlab function test_pi_flocking_gazebo/Translational Control2/Flocking1/MATLAB Function2 ==
  data: xi input; yi input; zi input; ui_gamma output; xr input; yr input; zr input; iep input size=3; ep output size=3; K_cts input

function [ui_gamma, ep] = naviFeedback(xi, yi, zi, xr, yr, zr, iep, K_cts)
    
    Kp = K_cts(1); Ki = K_cts(2);
    xmin = K_cts(3); xmax = K_cts(4);
       
    Pi = [xi ; yi ; zi] ;
    
    Pr = [xr ; yr ; zr] ;
    
    ep = Pi - Pr;
    
    ui_gamma = (-1).* satFcn(Kp.*(ep), xmin, xmax) + (-1).* satFcn(Ki.*(iep), xmin, xmax) ;
    
end

== matlab function test_pi_flocking_gazebo/Translational Control2/Flocking1/MATLAB Function3 ==
  data: xi input; yi input; zi input; vxi input; vyi input; vzi input; xobs parameter; yobs parameter; zobs parameter; vxobs parameter; vyobs parameter; vzobs parameter; phiBetanik output; R parameter; epsilon parameter; d_prime parameter; h parameter; bikobs output
function [phiBetanik, bikobs] = phiBetaFcn(xi, yi, zi, vxi, vyi, vzi, xobs, yobs, zobs, vxobs, vyobs, vzobs, R, epsilon, d_prime, h)
    
    dBeta = sigmaNormFun(d_prime, epsilon) ;
    
    Pi = [xi ; yi ; zi] ;
    Pc = [xobs ; yobs ; zobs] ;
    
    Vi = [vxi ; vyi ; vzi] ;
    Vc = [vxobs ; vyobs ; vzobs] ;

    % Compute closest point between the robot center and the obstacle
    % circumference (ossumming obstacles are circles)
    Pk = Pc + (Pi - Pc) * (R /norm(Pi - Pc)) ;
    %Pk = [xobs ; yobs] ;
    
    sigmaNormk = sigmaNormFun(Pk - Pi, epsilon) ;
    nik = gradSigmaFun(Pk - Pi, epsilon) ;
    
    sigma1k = sigma1Fun(sigmaNormk - dBeta) ;
    
    %% Position
    phiBetak = bumpFcn(sigmaNormk/dBeta,h) * (sigma1k - 1) ;
    phiBetanik = phiBetak.* nik ;
    
    %% Velocity
    bikobs = bumpFcn(sigmaNormk/dBeta,h).*(Vc + (Vi - Vc));
end

== matlab function test_pi_flocking_gazebo/Translational Control2/Flocking1/MATLAB Function4 ==
  data: xj input; yj input; zj input; vxj input; vyj input; vzj input; xk input; yk input; zk input; vxk input; vyk input; vzk input; xl input; yl input; zl input; vxl input; vyl input; vzl input; xobs parameter; yobs parameter; zobs parameter; phiBetaniknei output; R parameter; epsilon parameter; d_prime parameter; h parameter; vxobs parameter; vyobs parameter; vzobs parameter; bikve output
function [phiBetaniknei, bikve] = phiBetaFcn(xj, yj, zj, vxj, vyj, vzj, xk, yk, zk, vxk, vyk, vzk, xl, yl, zl, vxl, vyl, vzl, xobs, yobs, zobs, R, epsilon, d_prime, h, vxobs, vyobs, vzobs)
    
    dBeta = sigmaNormFun(d_prime, epsilon) ;
    
    Pj = [xj ; yj ; zj] ;
    Pk = [xk ; yk ; zk] ;
    Pl = [xl ; yl ; zl] ;
    Pc = [xobs ; yobs ; zobs] ;

    Vj = [vxj ; vyj ; vzj] ;
    Vk = [vxk ; vyk ; vzk] ;
    Vl = [vxl ; vyl ; vzl] ;
    Vc = [vxobs ; vyobs ; vzobs] ;

    % Compute closest point between the robot center and the obstacle
    % circumference (ossumming obstacles are circles)
    Pobsj = Pc + (Pj - Pc) * (R /norm(Pj - Pc)) ;
    Pobsk = Pc + (Pk - Pc) * (R /norm(Pk - Pc)) ;
    Pobsl = Pc + (Pl - Pc) * (R /norm(Pl - Pc)) ;
    %Pk = [xobs ; yobs] ;
    
    %%
    sigmaNormj = sigmaNormFun(Pobsj - Pj, epsilon) ;
    nij = gradSigmaFun(Pobsj - Pj, epsilon) ;
    
    sigmaNormk = sigmaNormFun(Pobsk - Pk, epsilon) ;
    nik = gradSigmaFun(Pobsk - Pk, epsilon) ;

    sigmaNorml = sigmaNormFun(Pobsl - Pl, epsilon) ;
    nil = gradSigmaFun(Pobsl - Pl, epsilon) ;

    %%
    sigma1j = sigma1Fun(sigmaNormj - dBeta) ;
    sigma1k = sigma1Fun(sigmaNormk - dBeta) ;
    sigma1l = sigma1Fun(sigmaNorml - dBeta) ;
            
    %%
    phiBetaj = bumpFcn(sigmaNormj/dBeta,h) * (sigma1j - 1) ;
    phiBetak = bumpFcn(sigmaNormk/dBeta,h) * (sigma1k - 1) ;
    phiBetal = bumpFcn(sigmaNorml/dBeta,h) * (sigma1l - 1) ;
            
    %% Position
    phiBetaniknei = phiBetaj.* nij + phiBetak.* nik + phiBetal.* nil;
    
    %% Velocity
    bikve = bumpFcn(sigmaNormj/dBeta,h).*(Vc + (Vj - Vc)) + bumpFcn(sigmaNormk/dBeta,h).*(Vc + (Vk - Vc)) + bumpFcn(sigmaNorml/dBeta,h).*(Vc + (Vl - Vc));
end

== matlab function test_pi_flocking_gazebo/Translational Control3/Flocking1/MATLAB Function ==
  data: xi input; yi input; zi input; phiAlpha output; xj input; yj input; zj input; xk input; yk input; zk input; xl input; yl input; zl input; params input

function phiAlpha  = phiAlphaFcn(xi, yi, zi, xj, yj, zj, xk, yk, zk, xl, yl, zl, params)
    
    % Flocking parameters
    epsilon = params(1); a = params(2); b = params(3); c = params(4); d = params(5); h = params(6);

    e = abs(a - b) / sqrt(4*a*b) ;

    cAlpha = sigmaNormFun(c, epsilon) ;
    dAlpha = sigmaNormFun(d, epsilon) ;

    %%
    Pi = [xi;yi;zi] ;
    Pj = [xj;yj;zj] ;
    Pk = [xk;yk;zk] ;
    Pl = [xl;yl;zl] ;

    %%
    sigmaNormj = sigmaNormFun(Pj - Pi, epsilon) ;
    nij = gradSigmaFun(Pj - Pi, epsilon) ;
    
    sigmaNormk = sigmaNormFun(Pk - Pi, epsilon) ;
    nik = gradSigmaFun(Pk - Pi, epsilon) ;

    sigmaNorml = sigmaNormFun(Pl - Pi, epsilon) ;
    nil = gradSigmaFun(Pl - Pi, epsilon) ;

    %%
    sigma1j = sigma1Fun(sigmaNormj - dAlpha + e) ;
    sigma1k = sigma1Fun(sigmaNormk - dAlpha + e) ;
    sigma1l = sigma1Fun(sigmaNorml - dAlpha + e) ;
            
    %% Position
    phiAlphaj = 0.5 * bumpFcn(sigmaNormj/cAlpha,h) * ((a+b)*sigma1j + (a-b)) ;
    phiAlphanij = phiAlphaj.* nij ;
    
    phiAlphak = 0.5 * bumpFcn(sigmaNormk/cAlpha,h) * ((a+b)*sigma1k + (a-b)) ;
    phiAlphanik = phiAlphak.* nik ;

    phiAlphal = 0.5 * bumpFcn(sigmaNorml/cAlpha,h) * ((a+b)*sigma1l + (a-b)) ;
    phiAlphanil = phiAlphal.* nil ;

    phiAlpha = phiAlphanij + phiAlphanik + phiAlphanil;

    
end

== matlab function test_pi_flocking_gazebo/Translational Control3/Flocking1/MATLAB Function1 ==
  data: phiAlpha input; phiAlpha_int input; ui_gamma input; yaw input; ieyaw input; Ui_pos output size=3; ui_yaw output; KP input; eyaw output

function [Ui_pos, ui_yaw, eyaw]  = ctrlLaw(phiAlpha, phiAlpha_int, ui_gamma, yaw, ieyaw, KP)  %, phiBetak, bikobs, phiBetanei, bikve
    
    % Control gains and parameters
    Kx = KP(1); Ky = KP(2); Kz = KP(3);
    Kix = KP(4); Kiy = KP(5); Kiz = KP(6);
    Kyaw = KP(8); Kiyaw = KP(7);
    
    hx_dot = Kx * phiAlpha(1,1) + Kix * phiAlpha_int(1,1) + ui_gamma(1,1);  %+ cBetax * (phiBetak(1,1) + phiBetanei(1,1)) + cdBetax * (bikobs(1,1) + bikve(1,1));
    hy_dot = Ky * phiAlpha(2,1) + Kiy * phiAlpha_int(2,1) + ui_gamma(2,1);  %+ cBetay * (phiBetak(2,1) + phiBetanei(2,1)) + cdBetay * (bikobs(2,1) + bikve(2,1));
    hz_dot = Kz * phiAlpha(3,1) + Kiz * phiAlpha_int(3,1) + ui_gamma(3,1);  %+ cBetaz * (phiBetak(3,1) + phiBetanei(3,1)) + cdBetaz * (bikobs(3,1) + bikve(3,1));
    

    eyaw = 0 - yaw;
    

    Ui_pos = [hx_dot; hy_dot; hz_dot] ;
    ui_yaw = Kyaw*eyaw + Kiyaw*ieyaw;

end

== matlab function test_pi_flocking_gazebo/Translational Control3/Flocking1/MATLAB Function2 ==
  data: xi input; yi input; zi input; ui_gamma output; xr input; yr input; zr input; iep input size=3; ep output size=3; K_cts input

function [ui_gamma, ep] = naviFeedback(xi, yi, zi, xr, yr, zr, iep, K_cts)
    
    Kp = K_cts(1); Ki = K_cts(2);
    xmin = K_cts(3); xmax = K_cts(4);
       
    Pi = [xi ; yi ; zi] ;
    
    Pr = [xr ; yr ; zr] ;
    
    ep = Pi - Pr;
    
    ui_gamma = (-1).* satFcn(Kp.*(ep), xmin, xmax) + (-1).* satFcn(Ki.*(iep), xmin, xmax) ;
    
end

== matlab function test_pi_flocking_gazebo/Translational Control3/Flocking1/MATLAB Function3 ==
  data: xi input; yi input; zi input; vxi input; vyi input; vzi input; xobs parameter; yobs parameter; zobs parameter; vxobs parameter; vyobs parameter; vzobs parameter; phiBetanik output; R parameter; epsilon parameter; d_prime parameter; h parameter; bikobs output
function [phiBetanik, bikobs] = phiBetaFcn(xi, yi, zi, vxi, vyi, vzi, xobs, yobs, zobs, vxobs, vyobs, vzobs, R, epsilon, d_prime, h)
    
    dBeta = sigmaNormFun(d_prime, epsilon) ;
    
    Pi = [xi ; yi ; zi] ;
    Pc = [xobs ; yobs ; zobs] ;
    
    Vi = [vxi ; vyi ; vzi] ;
    Vc = [vxobs ; vyobs ; vzobs] ;

    % Compute closest point between the robot center and the obstacle
    % circumference (ossumming obstacles are circles)
    Pk = Pc + (Pi - Pc) * (R /norm(Pi - Pc)) ;
    %Pk = [xobs ; yobs] ;
    
    sigmaNormk = sigmaNormFun(Pk - Pi, epsilon) ;
    nik = gradSigmaFun(Pk - Pi, epsilon) ;
    
    sigma1k = sigma1Fun(sigmaNormk - dBeta) ;
    
    %% Position
    phiBetak = bumpFcn(sigmaNormk/dBeta,h) * (sigma1k - 1) ;
    phiBetanik = phiBetak.* nik ;
    
    %% Velocity
    bikobs = bumpFcn(sigmaNormk/dBeta,h).*(Vc + (Vi - Vc));
end

== matlab function test_pi_flocking_gazebo/Translational Control3/Flocking1/MATLAB Function4 ==
  data: xj input; yj input; zj input; vxj input; vyj input; vzj input; xk input; yk input; zk input; vxk input; vyk input; vzk input; xl input; yl input; zl input; vxl input; vyl input; vzl input; xobs parameter; yobs parameter; zobs parameter; phiBetaniknei output; R parameter; epsilon parameter; d_prime parameter; h parameter; vxobs parameter; vyobs parameter; vzobs parameter; bikve output
function [phiBetaniknei, bikve] = phiBetaFcn(xj, yj, zj, vxj, vyj, vzj, xk, yk, zk, vxk, vyk, vzk, xl, yl, zl, vxl, vyl, vzl, xobs, yobs, zobs, R, epsilon, d_prime, h, vxobs, vyobs, vzobs)
    
    dBeta = sigmaNormFun(d_prime, epsilon) ;
    
    Pj = [xj ; yj ; zj] ;
    Pk = [xk ; yk ; zk] ;
    Pl = [xl ; yl ; zl] ;
    Pc = [xobs ; yobs ; zobs] ;

    Vj = [vxj ; vyj ; vzj] ;
    Vk = [vxk ; vyk ; vzk] ;
    Vl = [vxl ; vyl ; vzl] ;
    Vc = [vxobs ; vyobs ; vzobs] ;

    % Compute closest point between the robot center and the obstacle
    % circumference (ossumming obstacles are circles)
    Pobsj = Pc + (Pj - Pc) * (R /norm(Pj - Pc)) ;
    Pobsk = Pc + (Pk - Pc) * (R /norm(Pk - Pc)) ;
    Pobsl = Pc + (Pl - Pc) * (R /norm(Pl - Pc)) ;
    %Pk = [xobs ; yobs] ;
    
    %%
    sigmaNormj = sigmaNormFun(Pobsj - Pj, epsilon) ;
    nij = gradSigmaFun(Pobsj - Pj, epsilon) ;
    
    sigmaNormk = sigmaNormFun(Pobsk - Pk, epsilon) ;
    nik = gradSigmaFun(Pobsk - Pk, epsilon) ;

    sigmaNorml = sigmaNormFun(Pobsl - Pl, epsilon) ;
    nil = gradSigmaFun(Pobsl - Pl, epsilon) ;

    %%
    sigma1j = sigma1Fun(sigmaNormj - dBeta) ;
    sigma1k = sigma1Fun(sigmaNormk - dBeta) ;
    sigma1l = sigma1Fun(sigmaNorml - dBeta) ;
            
    %%
    phiBetaj = bumpFcn(sigmaNormj/dBeta,h) * (sigma1j - 1) ;
    phiBetak = bumpFcn(sigmaNormk/dBeta,h) * (sigma1k - 1) ;
    phiBetal = bumpFcn(sigmaNorml/dBeta,h) * (sigma1l - 1) ;
            
    %% Position
    phiBetaniknei = phiBetaj.* nij + phiBetak.* nik + phiBetal.* nil;
    
    %% Velocity
    bikve = bumpFcn(sigmaNormj/dBeta,h).*(Vc + (Vj - Vc)) + bumpFcn(sigmaNormk/dBeta,h).*(Vc + (Vk - Vc)) + bumpFcn(sigmaNorml/dBeta,h).*(Vc + (Vl - Vc));
end
